simulink model "TanqueFuzzy"  (R2017b)
settings: Solver=ode45  StartTime=0.0  StopTime=8  RelTol=1e-5  EnableMultiTasking=on
libraries: fuzblock x1
settings Model: Creator=Diego Santana  LastModifiedBy=D A Santana
settings DataIOCC: LimitDataPoints=on  SaveFormat=Array
settings OptimizationCC: LifeSpan=inf
settings DebuggingCC: SFUnexpectedBacktrackingDiag=warning  SFNoUnconditionalDefaultTransitionDiag=warning  SFExecutionAtInitializationDiag=none
settings HardwareCC: ProdBitPerPointer=32  ProdBitPerSizeT=32  ProdBitPerPtrDiffT=32  ProdLargestAtomicFloat=None  ProdIntDivRoundTo=Undefined  ProdEndianess=Unspecified  ProdWordSize=32  ProdHWDeviceType=32-bit Generic
settings ModelReferenceCC: PropagateSignalLabelsOutOfModel=off
settings CodeAppCC: StateflowObjectComments=on
settings GRTTargetCC: TargetLangStandard=C89/C90 (ANSI)  GeneratePreprocessorConditionals=Disable all
settings ConfigComp: CovMetricSettings=dw  CovHtmlReporting=on  CovSaveCumulativeToWorkspaceVar=on  CovSaveSingleToWorkspaceVar=on  CovExternalEMLEnable=off

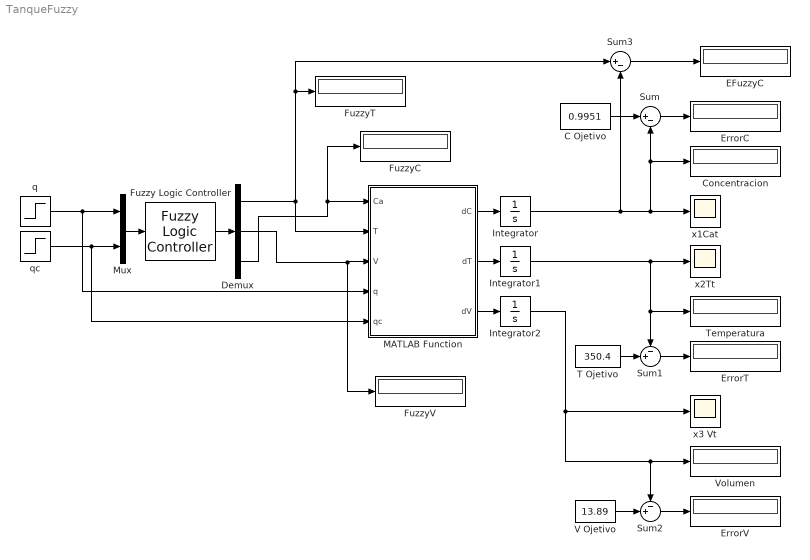
== system TanqueFuzzy ==
  C Ojetivo : Constant  Value=0.9951
  Concentracion : Display
  Demux : Demux  Outputs=3
  EFuzzyC : Display
  ErrorC : Display
  ErrorT : Display
  ErrorV : Display
  Fuzzy Logic Controller : fuzblock/Fuzzy Logic  Controller  FIS=reglasfuzzyfinaltabla  OutputSampleNumber=101  DataType=double  FuzzifiedInputs=off  RuleFiringStrengths=off  RuleOutputs=off  AggregatedOutputs=off  SimulateUsing=Interpreted execution
  FuzzyC : Display
  FuzzyT : Display
  FuzzyV : Display
  Integrator : Integrator  InitialCondition=0.9951
  Integrator1 : Integrator  InitialCondition=350.4
  Integrator2 : Integrator  InitialCondition=13.89
  MATLAB Function : MATLAB Function  TreatAsAtomicUnit=on
  Mux : Mux  Inputs=2
  Sum : Sum  Inputs=|+-
  Sum1 : Sum  Inputs=-+|
  Sum2 : Sum  Inputs=-+|
  Sum3 : Sum  Inputs=|+-
  T Ojetivo : Constant  Value=350.4
  Temperatura : Display
  V Ojetivo : Constant  Value=13.89
  Volumen : Display
  q : Step  Time=0  After=82  SampleTime=0
  qc : Step  Time=0  After=105  SampleTime=0
  x1Cat : Scope
  x2Tt : Scope
  x3 Vt : Scope
  wires:
  MATLAB Function/1(dC) -> Integrator/1
  MATLAB Function/2(dT) -> Integrator1/1
  MATLAB Function/3(dV) -> Integrator2/1
  Integrator1/1 -> Sum1/1, Temperatura/1, x2Tt/1
  Sum/1 -> ErrorC/1
  Integrator/1 -> Sum/2, Concentracion/1, x1Cat/1, Sum3/2
  C Ojetivo/1 -> Sum/1
  T Ojetivo/1 -> Sum1/2
  Sum1/1 -> ErrorT/1
  Sum2/1 -> ErrorV/1
  V Ojetivo/1 -> Sum2/2
  Integrator2/1 -> Sum2/1, Volumen/1, x3 Vt/1
  Fuzzy Logic Controller/1 -> Demux/1
  Mux/1 -> Fuzzy Logic Controller/1
  q/1 -> MATLAB Function/4(q), Mux/1
  qc/1 -> MATLAB Function/5(qc), Mux/2
  Demux/1 -> MATLAB Function/2(T), FuzzyT/1, Sum3/1
  Sum3/1 -> EFuzzyC/1
  Demux/2 -> MATLAB Function/3(V), FuzzyV/1
  Demux/3 -> FuzzyC/1, MATLAB Function/1(Ca)

== matlab function TanqueFuzzy/MATLAB Function ==
  data: Ca input; dC output; T input; V input; q input; qc input; dT output; dV output

function [dC,dT,dV] = tanqueCSTR (Ca,T,V,q,qc)
%Parámetros
Vt    =120;       %Volumen total 
To    =350;       %Temperatura del flujo entrada
Tco   =350;       %Temperatura del líquido refrigerante
deltH =-2e5;      %Calor de la reacción
Eact  =1e4;       %Energía de activación(E/R)
Cp    =1;         %Calores específicos
rho   =1e3;       %Densidad de los líquidos
ha    =7*10^5;    %Coeficiente de transferencia de calor
Cao   =1;         %Concentración de producto A en la alimentación del reactor
ko    =7.2e10;    %Constante de la velocidad de reacción
%Puntos de operacion personalizados
k4    =22;         %Constante de la válvula de salida del tanque
%q     =82;        %Flujo de Entrada q punto de operacion U1
%qc    =105;       %Flujo de Salida qc punto de operacion U2
%Ca    =0.9951;    %Concentracion Ca punto de operaxion X1
%T     =350.4;     %Tempratura T punto de operacion X2
%V     =13.89;     %Volumen V punto de operacion X3
k1    =(deltH*ko)/(rho*Cp);
k2    =(rho*Cp)/(rho*Cp);
k3    =ha/(rho*Cp);

%Ecuaciones que Modelan el Sistema
%Balance de Masas
    dC =(q/V*(Cao - Ca)) - (ko*Ca*exp(-Eact/T)); %expo revisar
%Balance de Energia
    dT =(q/V*(To - T)) + (k1*Ca*exp(-Eact/T)) + (k2*qc/V*(1-exp(-k3/qc))*(Tco-T));  
%Ecuacion Bernoulli
    dV =q-(k4*sqrt(V));
end
